simulink model "Cruise_Control_System"  (R2024a)
settings: Solver=VariableStepAuto  StartTime=0.0  StopTime=10.0  RelTol=1e-3
settings Model: Creator=VICTUS  LastModifiedBy=VICTUS

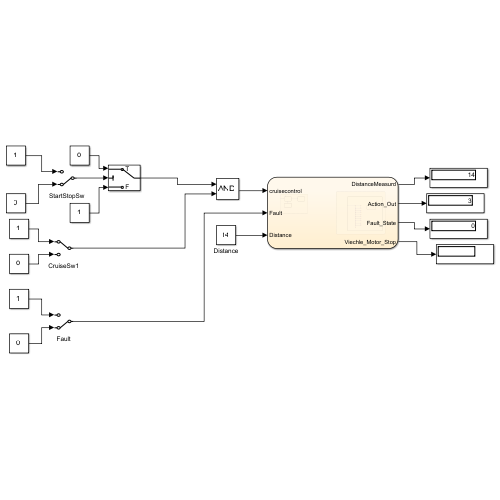
[thumbnail: Simulink's stored preview of the top-level diagram]
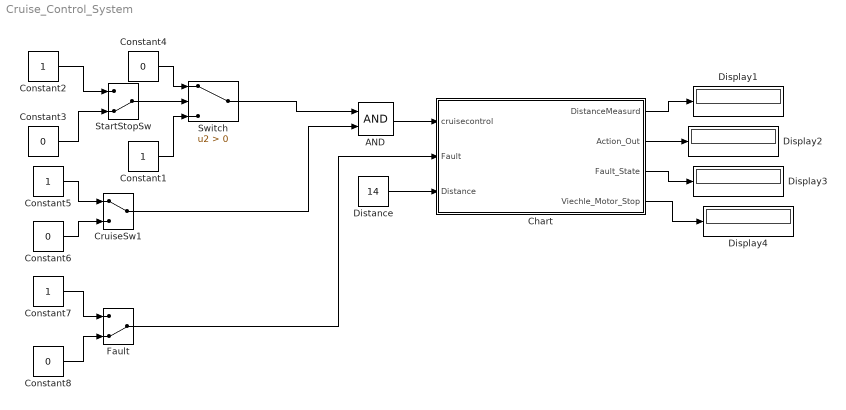
== system Cruise_Control_System ==
  AND : Logic  AllPortsSameDT=off  OutDataTypeStr=boolean
  Chart : Stateflow chart  TreatAsAtomicUnit=on
  Constant{1..2,5,7} (4 alike) : Constant  OutDataTypeStr=boolean
  Constant{3..4,6,8} (4 alike) : Constant  Value=0  OutDataTypeStr=boolean
  CruiseSw1 : ManualSwitch
  Display{1..4} (4 alike) : Display
  Distance : Constant  Value=14  OutDataTypeStr=double
  Fault : ManualSwitch  CurrentSetting=0
  StartStopSw : ManualSwitch  CurrentSetting=0
  Switch : Switch  Criteria=u2 > Threshold  SaturateOnIntegerOverflow=off  InputSameDT=off
  wires:
  Constant3/1 -> StartStopSw/2
  Constant2/1 -> StartStopSw/1
  StartStopSw/1 -> Switch/2
  Constant4/1 -> Switch/1
  Switch/1 -> AND/1
  Constant6/1 -> CruiseSw1/2
  Constant5/1 -> CruiseSw1/1
  Constant1/1 -> Switch/3
  Constant7/1 -> Fault/1
  Constant8/1 -> Fault/2
  Fault/1 -> Chart/2(Fault)
  AND/1 -> Chart/1(cruisecontrol)
  Distance/1 -> Chart/3(Distance)
  Chart/1(DistanceMeasurd) -> Display1/1
  Chart/2(Action_Out) -> Display2/1
  Chart/3(Fault_State) -> Display3/1
  CruiseSw1/1 -> AND/2
  Chart/4(Viechle_Motor_Stop) -> Display4/1

== stateflow chart Cruise_Control_System/Chart ==
  settings: executeAtInitialization=1
  state RegularSystem [parallel]
    settings: executionOrder=2
    state operation_of_cruise_control
      state DistanceMeasurd
        en:
        DistanceMeasurd = 10;
        DistanceMeasurd = Distance ;
        (history)
      operation_of_cruise_control -> (junction 34) : [cruisecontrol==1]
      (junction 34) -> (junction 36) [order 1] : [DistanceMeasurd > 15]
      (junction 34) -> (junction 40) [order 2]
      (junction 36) -> (junction 38) : {Action_Out = 2;}
          | %acclerate
      (junction 38) -> (junction 40)
      (junction 40) -> (junction 43)
      (junction 43) -> (junction 45) [order 1] : [DistanceMeasurd > 10]
      (junction 43) -> (junction 49) [order 2]
      (junction 45) -> (junction 47) : {Action_Out = 3;}
          | %decelrate
      (junction 47) -> (junction 49)
      (junction 49) -> (junction 53)
      (junction 53) -> (junction 55) [order 1] : [DistanceMeasurd > 5&& DistanceMeasurd < 10]
      (junction 53) -> (junction 59) [order 2]
      (junction 55) -> (junction 57) : {Action_Out = 1;}
          | %donothing
      (junction 57) -> (junction 59)
      (junction 59) -> (junction 63)
      (junction 63) -> (junction 65) [order 1] : [DistanceMeasurd < 5]
      (junction 63) -> (junction 69) [order 2]
      (junction 65) -> (junction 67) : {Action_Out = 4;}
          | %brake
      (junction 67) -> (junction 69)
      (junction 69) -> (junction 74)
      (junction 74) -> (junction 76) [order 1] : [DistanceMeasurd < 1.5]
      (junction 74) -> (junction 80) [order 2]
      (junction 76) -> (junction 78) : {Viechle_Motor_Stop = 1;}
      (junction 78) -> (junction 80)
      (junction 80) -> (junction 84)
  state FaultDetectionSystem [parallel]
    settings: executionOrder=1
    state FaultTimer
      en:
      Timer = 0;
      du:
      Timer = Timer + 1;
    state Notification
      en:
      Fault_State = 1;
    state Non_Fault
      en:
      Fault_State = 0;
    (default) -> FaultTimer
    FaultDetectionSystem -> FaultTimer : [Fault == 1]
    FaultTimer -> Notification [order 1] : [Timer == 10]
    FaultTimer -> Non_Fault [order 2] : [Timer <= 10]
  data: cruisecontrol input boolean; Fault input boolean; Distance input double; DistanceMeasurd output double; Timer local; Action_Out output double; Fault_State output double; Viechle_Motor_Stop output
